simulink model "kamerol"  (R2021b)
settings: Solver=VariableStepAuto  StartTime=0.0  StopTime=10.0  RelTol=1e-3
undefined symbols (not defined in the file): admireDB
libraries: simulink_extras x104, simulink x24, sharedutil x1
(part 6 of 14)

== system kamerol/Aerodynamics/RollMomentCoefficient/MachRegion4/Crmp ==
  in_bus : Inport
  Bus Selector : BusSelector  OutputSignals=AeroIn_Bus.angleOfAttack_deg,AeroIn_Bus.mach_nd,AeroIn_Bus.pc,AeroIn_Bus.qacorr
  Crmp_ : Subsystem
  Crmp : Outport
  wires:
  Bus Selector/4 -> Crmp_/4(qacorr)  "<qacorr>"
  Bus Selector/3 -> Crmp_/3(pc)  "<pc>"
  Bus Selector/2 -> Crmp_/2(mach_nd)  "<mach_nd>"
  Bus Selector/1 -> Crmp_/1(angleOfAttack_deg)  "<angleOfAttack_deg>"
  Crmp_/1(Crmp) -> Crmp/1
  in_bus/1 -> Bus Selector/1  "in_bus"

== system kamerol/Aerodynamics/RollMomentCoefficient/MachRegion4/Crmpbeta ==
  Crmpbeta_ : Constant  Value=0
  Crmpbeta : Outport
  wires:
  Crmpbeta_/1 -> Crmpbeta/1

== system kamerol/Aerodynamics/RollMomentCoefficient/MachRegion4/Crmr ==
  in_bus : Inport
  Bus Selector : BusSelector  OutputSignals=AeroIn_Bus.angleOfAttack_deg,AeroIn_Bus.mach_nd,AeroIn_Bus.rc
  Crmr_ : Subsystem
  Crmr : Outport
  wires:
  Bus Selector/3 -> Crmr_/3(rc)  "<rc>"
  Bus Selector/2 -> Crmr_/2(mach_nd)  "<mach_nd>"
  Bus Selector/1 -> Crmr_/1(angleOfAttack_deg)  "<angleOfAttack_deg>"
  Crmr_/1(Crmr) -> Crmr/1
  in_bus/1 -> Bus Selector/1  "in_bus"

== system kamerol/Aerodynamics/RollMomentCoefficient/MachRegion4/Crmrbeta ==
  Crmrbeta_ : Constant  Value=0
  Crmrbeta : Outport
  wires:
  Crmrbeta_/1 -> Crmrbeta/1

== system kamerol/Aerodynamics/RollMomentCoefficient/MachRegion4/Crmrde ==
  in_bus : Inport
  Bus Selector : BusSelector  OutputSignals=AeroIn_Bus.mach_nd,AeroIn_Bus.angleOfAttack_deg,AeroIn_Bus.rc,AeroIn_Bus.dEI,eieff,AeroIn_Bus.dEY,eoeff
  Crmrde_ : Subsystem
  Crmrde : Outport
  wires:
  Bus Selector/1 -> Crmrde_/1(mach_nd)  "<mach_nd>"
  Bus Selector/2 -> Crmrde_/2(angleOfAttack_deg)  "<angleOfAttack_deg>"
  Bus Selector/3 -> Crmrde_/3(rc)  "<rc>"
  Bus Selector/4 -> Crmrde_/4(dEI)  "<dEI>"
  Bus Selector/5 -> Crmrde_/5(eieff)  "<eieff>"
  Bus Selector/6 -> Crmrde_/6(dEY)  "<dEY>"
  Bus Selector/7 -> Crmrde_/7(eoeff)  "<eoeff>"
  Crmrde_/1(Crmrde) -> Crmrde/1
  in_bus/1 -> Bus Selector/1  "in_bus"

== system kamerol/Aerodynamics/RollMomentCoefficient/MachRegion4/eoeff1 ==
  AeroIn_Bus : Inport
  Bus Selector : BusSelector  OutputSignals=mach_nd
  CRMDAYOD_M : Lookup_n-D  NumberOfTableDimensions=1  BreakpointsForDimension1=admireDB.aerodata_asym_ext.CRMDAYOD.breakpoints.M  BreakpointsForDimension3=[5, 7]  Table=admireDB.aerodata_asym_ext.CRMDAYOD.newTable  ExtrapMethod=Clip  InternalRulePriority=Speed  RndMeth=Simplest  InputSameDT=on
  Constant : Constant
  Sum : Sum  Inputs=-+|
  eoeff : Outport
  eieff : Outport  Port=2
  wires:
  Sum/1 -> eieff/1
  CRMDAYOD_M/1 -> eoeff/1, Sum/1
  Constant/1 -> Sum/2
  Bus Selector/1 -> CRMDAYOD_M/1  "<mach_nd>"
  AeroIn_Bus/1 -> Bus Selector/1

== system kamerol/Aerodynamics/TangentialForceCoefficient/MachRegion1/Ctalfa ==
  in_bus : Inport
  Bus Selector : BusSelector  OutputSignals=AeroIn_Bus.angleOfAttack_deg
  CTAL_ALFA : Lookup_n-D  NumberOfTableDimensions=1  BreakpointsForDimension1=admireDB.aerodata_sym.CTAL.breakpoints.ALFA  BreakpointsForDimension3=[5, 7]  Table=admireDB.aerodata_sym.CTAL.newTable  ExtrapMethod=Clip  InternalRulePriority=Speed  RndMeth=Simplest  InputSameDT=on
  Ctalfa : Outport
  wires:
  Bus Selector/1 -> CTAL_ALFA/1  "<angleOfAttack_deg>"
  in_bus/1 -> Bus Selector/1
  CTAL_ALFA/1 -> Ctalfa/1  "Ctalfa"

== system kamerol/Aerodynamics/TangentialForceCoefficient/MachRegion1/Ctbasic ==
  in_bus : Inport
  Bus Selector : BusSelector  OutputSignals=AeroIn_Bus.mach_nd,AeroIn_Bus.altitude_m
  CTH_H_M : Lookup_n-D  BreakpointsForDimension1=admireDB.aerodata_sym.CTH.breakpoints.M  BreakpointsForDimension2=admireDB.aerodata_sym.CTH.breakpoints.H  BreakpointsForDimension3=[5, 7]  Table=admireDB.aerodata_sym.CTH.newTable  ExtrapMethod=Clip  InternalRulePriority=Speed  RndMeth=Simplest  InputSameDT=on
      settings: InputPortMap=u0,u1
  CTZERO_M : Lookup_n-D  NumberOfTableDimensions=1  BreakpointsForDimension1=admireDB.aerodata_sym.CTZERO.breakpoints.M  BreakpointsForDimension3=[5, 7]  Table=admireDB.aerodata_sym.CTZERO.newTable  ExtrapMethod=Clip  InternalRulePriority=Speed  RndMeth=Simplest  InputSameDT=on
  Constant : Constant  Value=1/1000
  Product : Product
  Sum1 : Sum  Inputs=|++
  Ctbasic : Outport
  wires:
  Sum1/1 -> Ctbasic/1
  CTZERO_M/1 -> Sum1/1
  CTH_H_M/1 -> Sum1/2
  Constant/1 -> Product/2
  Product/1 -> CTH_H_M/2
  Bus Selector/2 -> Product/1  "<altitude_m>"
  Bus Selector/1 -> CTZERO_M/1, CTH_H_M/1  "<mach_nd>"
  in_bus/1 -> Bus Selector/1  "in_bus"

== system kamerol/Aerodynamics/TangentialForceCoefficient/MachRegion1/Ctbeta ==
  in_bus : Inport
  Abs : Abs
  Bus Selector : BusSelector  OutputSignals=AeroIn_Bus.angleOfAttack_deg,AeroIn_Bus.dN,AeroIn_Bus.angleOfSideslip_deg
  CTBETA_DN_ALFA : Lookup_n-D  BreakpointsForDimension1=admireDB.aerodata_sym.CTBETA.breakpoints.ALFA  BreakpointsForDimension2=admireDB.aerodata_sym.CTBETA.breakpoints.DN  BreakpointsForDimension3=[5, 7]  Table=admireDB.aerodata_sym.CTBETA.newTable  ExtrapMethod=Clip  InternalRulePriority=Speed  RndMeth=Simplest  InputSameDT=on
      settings: InputPortMap=u0,u1
  CTKB_BETA : Lookup_n-D  NumberOfTableDimensions=1  BreakpointsForDimension1=admireDB.aerodata_sym.CTKB.breakpoints.BETA  BreakpointsForDimension3=[5, 7]  Table=admireDB.aerodata_sym.CTKB.newTable  ExtrapMethod=Clip  InternalRulePriority=Speed  RndMeth=Simplest  InputSameDT=on
  Product : Product
  Ctbeta : Outport
  wires:
  Product/1 -> Ctbeta/1
  CTBETA_DN_ALFA/1 -> Product/1
  CTKB_BETA/1 -> Product/2
  Abs/1 -> CTKB_BETA/1
  Bus Selector/3 -> Abs/1  "<angleOfSideslip_deg>"
  Bus Selector/1 -> CTBETA_DN_ALFA/1  "<angleOfAttack_deg>"
  Bus Selector/2 -> CTBETA_DN_ALFA/2  "<dN>"
  in_bus/1 -> Bus Selector/1

== system kamerol/Aerodynamics/TangentialForceCoefficient/MachRegion1/Ctda ==
  in_bus : Inport
  Abs : Abs
  Abs1 : Abs
  Abs2 : Abs
  Bus Selector : BusSelector  OutputSignals=AeroIn_Bus.angleOfAttack_deg,AeroIn_Bus.dAI,AeroIn_Bus.dAY
  Bus Selector1 : BusSelector  OutputSignals=eieff,eoeff
  CTDAAL_DA_ALFA : Lookup_n-D  BreakpointsForDimension1=admireDB.aerodata_sym.CTDAAL.breakpoints.ALFA  BreakpointsForDimension2=admireDB.aerodata_sym.CTDAAL.breakpoints.DA  BreakpointsForDimension3=[5, 7]  Table=admireDB.aerodata_sym.CTDAAL.newTable  ExtrapMethod=Clip  InternalRulePriority=Speed  RndMeth=Simplest  InputSameDT=on
      settings: InputPortMap=u0,u1
  CTDAAL_DA_ALFA1 : Lookup_n-D  BreakpointsForDimension1=admireDB.aerodata_sym.CTDAAL.breakpoints.ALFA  BreakpointsForDimension2=admireDB.aerodata_sym.CTDAAL.breakpoints.DA  BreakpointsForDimension3=[5, 7]  Table=admireDB.aerodata_sym.CTDAAL.newTable  ExtrapMethod=Clip  InternalRulePriority=Speed  RndMeth=Simplest  InputSameDT=on
      settings: InputPortMap=u0,u1
  Product : Product
  Product1 : Product
  Sum : Sum  Inputs=|++
  Ctda : Outport
  wires:
  Sum/1 -> Ctda/1
  Product1/1 -> Sum/2
  Product/1 -> Sum/1
  Bus Selector1/2 -> Product1/1  "<eoeff>"
  CTDAAL_DA_ALFA1/1 -> Product1/2
  Bus Selector1/1 -> Product/1  "<eieff>"
  CTDAAL_DA_ALFA/1 -> Product/2
  Abs2/1 -> CTDAAL_DA_ALFA1/2
  Abs1/1 -> CTDAAL_DA_ALFA/2
  Abs/1 -> CTDAAL_DA_ALFA/1, CTDAAL_DA_ALFA1/1
  Bus Selector/2 -> Abs1/1  "<dAI>"
  Bus Selector/1 -> Abs/1  "<angleOfAttack_deg>"
  in_bus/1 -> Bus Selector/1, Bus Selector1/1
  Bus Selector/3 -> Abs2/1  "<dAY>"

== system kamerol/Aerodynamics/TangentialForceCoefficient/MachRegion1/Ctdedn ==
  in_bus : Inport
  Bus Selector : BusSelector  OutputSignals=AeroIn_Bus.angleOfAttack_deg,AeroIn_Bus.dE,AeroIn_Bus.dN
  CTDNDE_ALFA_DE_DN : Lookup_n-D  NumberOfTableDimensions=3  BreakpointsForDimension1=admireDB.aerodata_sym.CTDNDE.breakpoints.ALFA  BreakpointsForDimension2=admireDB.aerodata_sym.CTDNDE.breakpoints.DE  BreakpointsForDimension3=admireDB.aerodata_sym.CTDNDE.breakpoints.DN  Table=admireDB.aerodata_sym.CTDNDE.newTable  ExtrapMethod=Clip  InternalRulePriority=Speed  RndMeth=Simplest  InputSameDT=on
      settings: InputPortMap=u0,u1,u2
  Ctdedn : Outport
  wires:
  Bus Selector/1 -> CTDNDE_ALFA_DE_DN/1  "<angleOfAttack_deg>"
  Bus Selector/3 -> CTDNDE_ALFA_DE_DN/3  "<dN>"
  CTDNDE_ALFA_DE_DN/1 -> Ctdedn/1
  Bus Selector/2 -> CTDNDE_ALFA_DE_DN/2  "<dE>"
  in_bus/1 -> Bus Selector/1

== system kamerol/Aerodynamics/TangentialForceCoefficient/MachRegion1/Ctdei ==
  in_bus : Inport
  Bus Selector : BusSelector  OutputSignals=AeroIn_Bus.angleOfAttack_deg,AeroIn_Bus.dEI,eieff
  CTDEAL_DE_ALFA : Lookup_n-D  BreakpointsForDimension1=admireDB.aerodata_sym.CTDEAL.breakpoints.ALFA  BreakpointsForDimension2=admireDB.aerodata_sym.CTDEAL.breakpoints.DE  BreakpointsForDimension3=[5, 7]  Table=admireDB.aerodata_sym.CTDEAL.newTable  ExtrapMethod=Clip  InternalRulePriority=Speed  RndMeth=Simplest  InputSameDT=on
      settings: InputPortMap=u0,u1
  Product : Product
  Ctdei : Outport
  wires:
  Product/1 -> Ctdei/1
  Bus Selector/3 -> Product/2  "<eieff>"
  CTDEAL_DE_ALFA/1 -> Product/1
  Bus Selector/1 -> CTDEAL_DE_ALFA/1  "<angleOfAttack_deg>"
  Bus Selector/2 -> CTDEAL_DE_ALFA/2  "<dEI>"
  in_bus/1 -> Bus Selector/1

== system kamerol/Aerodynamics/TangentialForceCoefficient/MachRegion1/Ctdey ==
  in_bus : Inport
  Bus Selector : BusSelector  OutputSignals=AeroIn_Bus.angleOfAttack_deg,AeroIn_Bus.dEY,eoeff
  CTDEAL_DE_ALFA : Lookup_n-D  BreakpointsForDimension1=admireDB.aerodata_sym.CTDEAL.breakpoints.ALFA  BreakpointsForDimension2=admireDB.aerodata_sym.CTDEAL.breakpoints.DE  BreakpointsForDimension3=[5, 7]  Table=admireDB.aerodata_sym.CTDEAL.newTable  ExtrapMethod=Clip  InternalRulePriority=Speed  RndMeth=Simplest  InputSameDT=on
      settings: InputPortMap=u0,u1
  Product : Product
  Ctdey : Outport
  wires:
  in_bus/1 -> Bus Selector/1
  Bus Selector/2 -> CTDEAL_DE_ALFA/2  "<dEY>"
  Bus Selector/1 -> CTDEAL_DE_ALFA/1  "<angleOfAttack_deg>"
  CTDEAL_DE_ALFA/1 -> Product/1
  Bus Selector/3 -> Product/2  "<eoeff>"
  Product/1 -> Ctdey/1

== system kamerol/Aerodynamics/TangentialForceCoefficient/MachRegion1/Ctdle ==
  in_bus : Inport
  Bus Selector : BusSelector  OutputSignals=AeroIn_Bus.angleOfAttack_deg,AeroIn_Bus.lef_deg,AeroIn_Bus.dN
  CTDLEAL_DLE_ALFA : Lookup_n-D  BreakpointsForDimension1=admireDB.aerodata_sym.CTDLEAL.breakpoints.ALFA  BreakpointsForDimension2=admireDB.aerodata_sym.CTDLEAL.breakpoints.DLE  BreakpointsForDimension3=[5, 7]  Table=admireDB.aerodata_sym.CTDLEAL.newTable  ExtrapMethod=Clip  InternalRulePriority=Speed  RndMeth=Simplest  InputSameDT=on
      settings: InputPortMap=u0,u1
  CTLEDNAL_DN_ALFA : Lookup_n-D  BreakpointsForDimension1=admireDB.aerodata_sym.CTLEDNAL.breakpoints.ALFA  BreakpointsForDimension2=admireDB.aerodata_sym.CTLEDNAL.breakpoints.DN  BreakpointsForDimension3=[5, 7]  Table=admireDB.aerodata_sym.CTLEDNAL.newTable  ExtrapMethod=Clip  InternalRulePriority=Speed  RndMeth=Simplest  InputSameDT=on
      settings: InputPortMap=u0,u1
  Constant : Constant  Value=1/27
  Product : Product  Inputs=3
  Sum : Sum  Inputs=|++
  Ctdle : Outport
  wires:
  Product/1 -> Sum/2
  Constant/1 -> Product/3
  CTLEDNAL_DN_ALFA/1 -> Product/1
  Bus Selector/3 -> CTLEDNAL_DN_ALFA/2  "<dN>"
  Sum/1 -> Ctdle/1
  Bus Selector/1 -> CTLEDNAL_DN_ALFA/1, CTDLEAL_DLE_ALFA/1  "<angleOfAttack_deg>"
  Bus Selector/2 -> Product/2, CTDLEAL_DLE_ALFA/2  "<lef_deg>"
  CTDLEAL_DLE_ALFA/1 -> Sum/1
  in_bus/1 -> Bus Selector/1

== system kamerol/Aerodynamics/TangentialForceCoefficient/MachRegion1/Ctdn ==
  in_bus : Inport
  Bus Selector : BusSelector  OutputSignals=AeroIn_Bus.angleOfAttack_deg,AeroIn_Bus.dN
  CTDNAL_DN_ALFA : Lookup_n-D  BreakpointsForDimension1=admireDB.aerodata_sym.CTDNAL.breakpoints.ALFA  BreakpointsForDimension2=admireDB.aerodata_sym.CTDNAL.breakpoints.DN  BreakpointsForDimension3=[5, 7]  Table=admireDB.aerodata_sym.CTDNAL.newTable  ExtrapMethod=Clip  InternalRulePriority=Speed  RndMeth=Simplest  InputSameDT=on
      settings: InputPortMap=u0,u1
  Ctdn : Outport
  wires:
  in_bus/1 -> Bus Selector/1
  CTDNAL_DN_ALFA/1 -> Ctdn/1
  Bus Selector/2 -> CTDNAL_DN_ALFA/2  "<dN>"
  Bus Selector/1 -> CTDNAL_DN_ALFA/1  "<angleOfAttack_deg>"

== system kamerol/Aerodynamics/TangentialForceCoefficient/MachRegion1/Ctdr ==
  in_bus : Inport
  Abs : Abs
  Bus Selector : BusSelector  OutputSignals=AeroIn_Bus.mach_nd,AeroIn_Bus.rud_deg
  CTMDR_DR_M : Lookup_n-D  BreakpointsForDimension1=admireDB.aerodata_sym.CTMDR.breakpoints.M  BreakpointsForDimension2=admireDB.aerodata_sym.CTMDR.breakpoints.DR  BreakpointsForDimension3=[5, 7]  Table=admireDB.aerodata_sym.CTMDR.newTable  ExtrapMethod=Clip  InternalRulePriority=Speed  RndMeth=Simplest  InputSameDT=on
      settings: InputPortMap=u0,u1
  Ctdr : Outport
  wires:
  Abs/1 -> CTMDR_DR_M/2
  Bus Selector/1 -> CTMDR_DR_M/1  "<mach_nd>"
  Bus Selector/2 -> Abs/1  "<rud_deg>"
  in_bus/1 -> Bus Selector/1
  CTMDR_DR_M/1 -> Ctdr/1

== system kamerol/Aerodynamics/TangentialForceCoefficient/MachRegion1/Cthigh ==
  in_bus : Inport
  Bus Selector : BusSelector  OutputSignals=AeroIn_Bus.angleOfAttack_deg,AeroIn_Bus.dN,AeroIn_Bus.dE
  CTHDE_DE_ALFA : Lookup_n-D  BreakpointsForDimension1=admireDB.aerodata_high.CTHDE.breakpoints.ALFA  BreakpointsForDimension2=admireDB.aerodata_high.CTHDE.breakpoints.DE  BreakpointsForDimension3=[5, 7]  Table=admireDB.aerodata_high.CTHDE.newTable  ExtrapMethod=Clip  InternalRulePriority=Speed  RndMeth=Simplest  InputSameDT=on
      settings: InputPortMap=u0,u1
  CTHDN_DN_ALFA : Lookup_n-D  BreakpointsForDimension1=admireDB.aerodata_high.CTHDN.breakpoints.ALFA  BreakpointsForDimension2=admireDB.aerodata_high.CTHDN.breakpoints.DN  BreakpointsForDimension3=[5, 7]  Table=admireDB.aerodata_high.CTHDN.newTable  ExtrapMethod=Clip  InternalRulePriority=Speed  RndMeth=Simplest  InputSameDT=on
      settings: InputPortMap=u0,u1
  CTHZERO_ALFA : Lookup_n-D  NumberOfTableDimensions=1  BreakpointsForDimension1=admireDB.aerodata_high.CTHZERO.breakpoints.ALFA  BreakpointsForDimension3=[5, 7]  Table=admireDB.aerodata_high.CTHZERO.newTable  ExtrapMethod=Clip  InternalRulePriority=Speed  RndMeth=Simplest  InputSameDT=on
  Sum : Sum  Inputs=+++
  Cthigh : Outport
  wires:
  CTHZERO_ALFA/1 -> Sum/1
  CTHDE_DE_ALFA/1 -> Sum/3
  CTHDN_DN_ALFA/1 -> Sum/2
  Bus Selector/3 -> CTHDE_DE_ALFA/2  "<dE>"
  Bus Selector/2 -> CTHDN_DN_ALFA/2  "<dN>"
  Sum/1 -> Cthigh/1
  in_bus/1 -> Bus Selector/1
  Bus Selector/1 -> CTHZERO_ALFA/1, CTHDN_DN_ALFA/1, CTHDE_DE_ALFA/1  "<angleOfAttack_deg>"

== system kamerol/Aerodynamics/TangentialForceCoefficient/MachRegion1/Ctlg ==
  in_bus : Inport
  Abs : Abs
  Bus Selector : BusSelector  OutputSignals=AeroIn_Bus.angleOfAttack_deg,AeroIn_Bus.angleOfSideslip_deg,AeroIn_Bus.lg_bool
  CTLST_BETA_ALFA : Lookup_n-D  BreakpointsForDimension1=admireDB.aerodata_sym.CTLST.breakpoints.ALFA  BreakpointsForDimension2=admireDB.aerodata_sym.CTLST.breakpoints.BETA  BreakpointsForDimension3=[5, 7]  Table=admireDB.aerodata_sym.CTLST.newTable  ExtrapMethod=Clip  InternalRulePriority=Speed  RndMeth=Simplest  InputSameDT=on
      settings: InputPortMap=u0,u1
  Product : Product  Inputs=**
  Ctlg : Outport
  wires:
  Abs/1 -> CTLST_BETA_ALFA/2
  Bus Selector/3 -> Product/2  "<lg_bool>"
  CTLST_BETA_ALFA/1 -> Product/1
  in_bus/1 -> Bus Selector/1
  Bus Selector/2 -> Abs/1  "<angleOfSideslip_deg>"
  Bus Selector/1 -> CTLST_BETA_ALFA/1  "<angleOfAttack_deg>"
  Product/1 -> Ctlg/1

== system kamerol/Aerodynamics/TangentialForceCoefficient/MachRegion1/eoeff ==
  AeroIn_Bus : Inport
  Bus Selector : BusSelector  OutputSignals=mach_nd
  CTDEYODE_M : Lookup_n-D  NumberOfTableDimensions=1  BreakpointsForDimension1=admireDB.aerodata_sym.CTDEYODE.breakpoints.M  BreakpointsForDimension3=[5, 7]  Table=admireDB.aerodata_sym.CTDEYODE.newTable  ExtrapMethod=Clip  InternalRulePriority=Speed  RndMeth=Simplest  InputSameDT=on
  Constant : Constant
  Sum : Sum  Inputs=-+|
  eoeff : Outport
  eieff : Outport  Port=2
  wires:
  Sum/1 -> eieff/1
  CTDEYODE_M/1 -> eoeff/1, Sum/1
  Constant/1 -> Sum/2
  Bus Selector/1 -> CTDEYODE_M/1  "<mach_nd>"
  AeroIn_Bus/1 -> Bus Selector/1

== system kamerol/Aerodynamics/TangentialForceCoefficient/MachRegion2/Ctalfa ==
  in_bus : Inport
  Bus Selector : BusSelector  OutputSignals=AeroIn_Bus.angleOfAttack_deg,AeroIn_Bus.tflow,AeroIn_Bus.tfhigh
  CTAL_ALFA : Lookup_n-D  NumberOfTableDimensions=1  BreakpointsForDimension1=admireDB.aerodata_sym.CTAL.breakpoints.ALFA  BreakpointsForDimension3=[5, 7]  Table=admireDB.aerodata_sym.CTAL.newTable  ExtrapMethod=Clip  InternalRulePriority=Speed  RndMeth=Simplest  InputSameDT=on
  CTMA_M_ALFA : Lookup_n-D  BreakpointsForDimension1=admireDB.aerodata_sym.CTMA.breakpoints.ALFA  BreakpointsForDimension2=admireDB.aerodata_sym.CTMA.breakpoints.M  BreakpointsForDimension3=[5, 7]  Table=admireDB.aerodata_sym.CTMA.newTable  ExtrapMethod=Clip  InternalRulePriority=Speed  RndMeth=Simplest  InputSameDT=on
      settings: InputPortMap=u0,u1
  Constant : Constant  Value=0.5
  Product : Product
  Product1 : Product
  Sum : Sum  Inputs=|++
  Ctalfa : Outport
  wires:
  Bus Selector/3 -> Product1/1  "<tfhigh>"
  Bus Selector/2 -> Product/2  "<tflow>"
  Product1/1 -> Sum/2
  CTMA_M_ALFA/1 -> Product1/2
  Sum/1 -> Ctalfa/1
  Product/1 -> Sum/1
  Constant/1 -> CTMA_M_ALFA/2
  CTAL_ALFA/1 -> Product/1  "Ctalfa"
  in_bus/1 -> Bus Selector/1
  Bus Selector/1 -> CTAL_ALFA/1, CTMA_M_ALFA/1  "<angleOfAttack_deg>"

== system kamerol/Aerodynamics/TangentialForceCoefficient/MachRegion2/Ctbasic ==
  in_bus : Inport
  Bus Selector : BusSelector  OutputSignals=AeroIn_Bus.mach_nd,AeroIn_Bus.altitude_m
  CTH_H_M : Lookup_n-D  BreakpointsForDimension1=admireDB.aerodata_sym.CTH.breakpoints.M  BreakpointsForDimension2=admireDB.aerodata_sym.CTH.breakpoints.H  BreakpointsForDimension3=[5, 7]  Table=admireDB.aerodata_sym.CTH.newTable  ExtrapMethod=Clip  InternalRulePriority=Speed  RndMeth=Simplest  InputSameDT=on
      settings: InputPortMap=u0,u1
  CTZERO_M : Lookup_n-D  NumberOfTableDimensions=1  BreakpointsForDimension1=admireDB.aerodata_sym.CTZERO.breakpoints.M  BreakpointsForDimension3=[5, 7]  Table=admireDB.aerodata_sym.CTZERO.newTable  ExtrapMethod=Clip  InternalRulePriority=Speed  RndMeth=Simplest  InputSameDT=on
  Constant : Constant  Value=1/1000
  Product : Product
  Sum1 : Sum  Inputs=|++
  Ctbasic : Outport
  wires:
  CTH_H_M/1 -> Sum1/2
  Constant/1 -> Product/2
  Bus Selector/2 -> Product/1  "<altitude_m>"
  Product/1 -> CTH_H_M/2
  CTZERO_M/1 -> Sum1/1
  Bus Selector/1 -> CTZERO_M/1, CTH_H_M/1  "<mach_nd>"
  in_bus/1 -> Bus Selector/1  "in_bus"
  Sum1/1 -> Ctbasic/1

== system kamerol/Aerodynamics/TangentialForceCoefficient/MachRegion2/Ctbeta ==
  in_bus : Inport
  Abs : Abs
  Bus Selector : BusSelector  OutputSignals=AeroIn_Bus.angleOfAttack_deg,AeroIn_Bus.dN,AeroIn_Bus.tflow,AeroIn_Bus.angleOfSideslip_deg
  CTBETA_DN_ALFA : Lookup_n-D  BreakpointsForDimension1=admireDB.aerodata_sym.CTBETA.breakpoints.ALFA  BreakpointsForDimension2=admireDB.aerodata_sym.CTBETA.breakpoints.DN  BreakpointsForDimension3=[5, 7]  Table=admireDB.aerodata_sym.CTBETA.newTable  ExtrapMethod=Clip  InternalRulePriority=Speed  RndMeth=Simplest  InputSameDT=on
      settings: InputPortMap=u0,u1
  CTKB_BETA : Lookup_n-D  NumberOfTableDimensions=1  BreakpointsForDimension1=admireDB.aerodata_sym.CTKB.breakpoints.BETA  BreakpointsForDimension3=[5, 7]  Table=admireDB.aerodata_sym.CTKB.newTable  ExtrapMethod=Clip  InternalRulePriority=Speed  RndMeth=Simplest  InputSameDT=on
  Product : Product  Inputs=3
  Ctbeta : Outport
  wires:
  Bus Selector/3 -> Product/2  "<tflow>"
  in_bus/1 -> Bus Selector/1
  Bus Selector/2 -> CTBETA_DN_ALFA/2  "<dN>"
  Bus Selector/1 -> CTBETA_DN_ALFA/1  "<angleOfAttack_deg>"
  Bus Selector/4 -> Abs/1  "<angleOfSideslip_deg>"
  Abs/1 -> CTKB_BETA/1
  CTKB_BETA/1 -> Product/3
  CTBETA_DN_ALFA/1 -> Product/1
  Product/1 -> Ctbeta/1

== system kamerol/Aerodynamics/TangentialForceCoefficient/MachRegion2/Ctda ==
  in_bus : Inport
  Abs : Abs
  Abs1 : Abs
  Abs2 : Abs
  Bus Selector : BusSelector  OutputSignals=AeroIn_Bus.angleOfAttack_deg,AeroIn_Bus.dAI,AeroIn_Bus.dAY
  Bus Selector1 : BusSelector  OutputSignals=AeroIn_Bus.tflow,eiefflow,eoefflow,eieffhigh,eoeffhigh,AeroIn_Bus.tfhigh
  CTDAAL_DA_ALFA : Lookup_n-D  BreakpointsForDimension1=admireDB.aerodata_sym.CTDAAL.breakpoints.ALFA  BreakpointsForDimension2=admireDB.aerodata_sym.CTDAAL.breakpoints.DA  BreakpointsForDimension3=[5, 7]  Table=admireDB.aerodata_sym.CTDAAL.newTable  ExtrapMethod=Clip  InternalRulePriority=Speed  RndMeth=Simplest  InputSameDT=on
      settings: InputPortMap=u0,u1
  CTDAAL_DA_ALFA1 : Lookup_n-D  BreakpointsForDimension1=admireDB.aerodata_sym.CTDAAL.breakpoints.ALFA  BreakpointsForDimension2=admireDB.aerodata_sym.CTDAAL.breakpoints.DA  BreakpointsForDimension3=[5, 7]  Table=admireDB.aerodata_sym.CTDAAL.newTable  ExtrapMethod=Clip  InternalRulePriority=Speed  RndMeth=Simplest  InputSameDT=on
      settings: InputPortMap=u0,u1
  CTDAM_DA_M : Lookup_n-D  BreakpointsForDimension1=admireDB.aerodata_sym.CTDAM.breakpoints.M  BreakpointsForDimension2=admireDB.aerodata_sym.CTDAM.breakpoints.DA  BreakpointsForDimension3=[5, 7]  Table=admireDB.aerodata_sym.CTDAM.newTable  ExtrapMethod=Clip  InternalRulePriority=Speed  RndMeth=Simplest  InputSameDT=on
      settings: InputPortMap=u0,u1
  CTDAM_DA_M1 : Lookup_n-D  BreakpointsForDimension1=admireDB.aerodata_sym.CTDAM.breakpoints.M  BreakpointsForDimension2=admireDB.aerodata_sym.CTDAM.breakpoints.DA  BreakpointsForDimension3=[5, 7]  Table=admireDB.aerodata_sym.CTDAM.newTable  ExtrapMethod=Clip  InternalRulePriority=Speed  RndMeth=Simplest  InputSameDT=on
      settings: InputPortMap=u0,u1
  Product{,1..5} (6 alike) : Product
  Sum : Sum  Inputs=|++
  Sum1 : Sum  Inputs=++|
  Sum2 : Sum  Inputs=|++
  mach_nd_cnst : Constant  Value=0.5
  Ctda : Outport
  wires:
  Product5/1 -> Sum1/2
  Bus Selector1/6 -> Product5/1  "<tfhigh>"
  Sum2/1 -> Product5/2
  Product3/1 -> Sum2/2
  Product4/1 -> Sum2/1
  Bus Selector1/5 -> Product3/1  "<eoeffhigh>"
  Bus Selector1/4 -> Product4/1  "<eieffhigh>"
  CTDAM_DA_M/1 -> Product4/2
  CTDAM_DA_M1/1 -> Product3/2
  mach_nd_cnst/1 -> CTDAM_DA_M/1, CTDAM_DA_M1/1
  Sum1/1 -> Ctda/1
  Product2/1 -> Sum1/1
  Bus Selector1/1 -> Product2/1  "<tflow>"
  Bus Selector/3 -> Abs2/1  "<dAY>"
  in_bus/1 -> Bus Selector1/1, Bus Selector/1
  Bus Selector/1 -> Abs/1  "<angleOfAttack_deg>"
  Bus Selector/2 -> Abs1/1  "<dAI>"
  Abs/1 -> CTDAAL_DA_ALFA/1, CTDAAL_DA_ALFA1/1
  Abs1/1 -> CTDAAL_DA_ALFA/2, CTDAM_DA_M/2
  Abs2/1 -> CTDAAL_DA_ALFA1/2, CTDAM_DA_M1/2
  CTDAAL_DA_ALFA/1 -> Product/2
  Bus Selector1/2 -> Product/1  "<eiefflow>"
  CTDAAL_DA_ALFA1/1 -> Product1/2
  Bus Selector1/3 -> Product1/1  "<eoefflow>"
  Product/1 -> Sum/1
  Product1/1 -> Sum/2
  Sum/1 -> Product2/2

== system kamerol/Aerodynamics/TangentialForceCoefficient/MachRegion2/Ctdedn ==
  in_bus : Inport
  Bus Selector : BusSelector  OutputSignals=AeroIn_Bus.angleOfAttack_deg,AeroIn_Bus.dE,AeroIn_Bus.dN,AeroIn_Bus.tflow
  CTDNDE_ALFA_DE_DN1 : Lookup_n-D  NumberOfTableDimensions=3  BreakpointsForDimension1=admireDB.aerodata_sym.CTDNDE.breakpoints.ALFA  BreakpointsForDimension2=admireDB.aerodata_sym.CTDNDE.breakpoints.DE  BreakpointsForDimension3=admireDB.aerodata_sym.CTDNDE.breakpoints.DN  Table=admireDB.aerodata_sym.CTDNDE.newTable  ExtrapMethod=Clip  InternalRulePriority=Speed  RndMeth=Simplest  InputSameDT=on
      settings: InputPortMap=u0,u1,u2
  Product : Product
  Ctdedn : Outport
  wires:
  Bus Selector/4 -> Product/2  "<tflow>"
  Product/1 -> Ctdedn/1
  Bus Selector/1 -> CTDNDE_ALFA_DE_DN1/1  "<angleOfAttack_deg>"
  Bus Selector/3 -> CTDNDE_ALFA_DE_DN1/3  "<dN>"
  Bus Selector/2 -> CTDNDE_ALFA_DE_DN1/2  "<dE>"
  in_bus/1 -> Bus Selector/1
  CTDNDE_ALFA_DE_DN1/1 -> Product/1

== system kamerol/Aerodynamics/TangentialForceCoefficient/MachRegion2/Ctdei ==
  in_bus : Inport
  Bus Selector : BusSelector  OutputSignals=AeroIn_Bus.angleOfAttack_deg,AeroIn_Bus.dEI,eiefflow,AeroIn_Bus.tflow,eieffhigh,AeroIn_Bus.tfhigh
  CTDEAL_DE_ALFA1 : Lookup_n-D  BreakpointsForDimension1=admireDB.aerodata_sym.CTDEAL.breakpoints.ALFA  BreakpointsForDimension2=admireDB.aerodata_sym.CTDEAL.breakpoints.DE  BreakpointsForDimension3=[5, 7]  Table=admireDB.aerodata_sym.CTDEAL.newTable  ExtrapMethod=Clip  InternalRulePriority=Speed  RndMeth=Simplest  InputSameDT=on
      settings: InputPortMap=u0,u1
  CTMDEA_ALFA_DE_M : Lookup_n-D  NumberOfTableDimensions=3  BreakpointsForDimension1=admireDB.aerodata_sym.CTMDEA.breakpoints.ALFA  BreakpointsForDimension2=admireDB.aerodata_sym.CTMDEA.breakpoints.DE  BreakpointsForDimension3=admireDB.aerodata_sym.CTMDEA.breakpoints.M  Table=admireDB.aerodata_sym.CTMDEA.newTable  ExtrapMethod=Clip  InternalRulePriority=Speed  RndMeth=Simplest  InputSameDT=on
      settings: InputPortMap=u0,u1,u2
  Product : Product  Inputs=3
  Product1 : Product  Inputs=3
  Sum : Sum  Inputs=|++
  mach_nd_cnst : Constant  Value=0.5
  Ctdei : Outport
  wires:
  Product1/1 -> Sum/2
  Sum/1 -> Ctdei/1
  Bus Selector/6 -> Product1/2  "<tfhigh>"
  CTMDEA_ALFA_DE_M/1 -> Product1/3
  Bus Selector/5 -> Product1/1  "<eieffhigh>"
  Bus Selector/4 -> Product/3  "<tflow>"
  mach_nd_cnst/1 -> CTMDEA_ALFA_DE_M/3
  in_bus/1 -> Bus Selector/1
  Bus Selector/2 -> CTMDEA_ALFA_DE_M/2, CTDEAL_DE_ALFA1/2  "<dEI>"
  Bus Selector/1 -> CTDEAL_DE_ALFA1/1, CTMDEA_ALFA_DE_M/1  "<angleOfAttack_deg>"
  CTDEAL_DE_ALFA1/1 -> Product/1
  Bus Selector/3 -> Product/2  "<eiefflow>"
  Product/1 -> Sum/1

== system kamerol/Aerodynamics/TangentialForceCoefficient/MachRegion2/Ctdey ==
  in_bus : Inport
  Bus Selector : BusSelector  OutputSignals=AeroIn_Bus.angleOfAttack_deg,AeroIn_Bus.dEY,eoefflow,AeroIn_Bus.tflow,eoeffhigh,AeroIn_Bus.tfhigh
  CTDEAL_DE_ALFA1 : Lookup_n-D  BreakpointsForDimension1=admireDB.aerodata_sym.CTDEAL.breakpoints.ALFA  BreakpointsForDimension2=admireDB.aerodata_sym.CTDEAL.breakpoints.DE  BreakpointsForDimension3=[5, 7]  Table=admireDB.aerodata_sym.CTDEAL.newTable  ExtrapMethod=Clip  InternalRulePriority=Speed  RndMeth=Simplest  InputSameDT=on
      settings: InputPortMap=u0,u1
  CTMDEA_ALFA_DE_M : Lookup_n-D  NumberOfTableDimensions=3  BreakpointsForDimension1=admireDB.aerodata_sym.CTMDEA.breakpoints.ALFA  BreakpointsForDimension2=admireDB.aerodata_sym.CTMDEA.breakpoints.DE  BreakpointsForDimension3=admireDB.aerodata_sym.CTMDEA.breakpoints.M  Table=admireDB.aerodata_sym.CTMDEA.newTable  ExtrapMethod=Clip  InternalRulePriority=Speed  RndMeth=Simplest  InputSameDT=on
      settings: InputPortMap=u0,u1,u2
  Product : Product  Inputs=3
  Product1 : Product  Inputs=3
  Sum : Sum  Inputs=|++
  mach_nd_cnst : Constant  Value=0.5
  Ctdey : Outport
  wires:
  Product/1 -> Sum/1
  Bus Selector/3 -> Product/2  "<eoefflow>"
  CTDEAL_DE_ALFA1/1 -> Product/1
  Bus Selector/1 -> CTDEAL_DE_ALFA1/1, CTMDEA_ALFA_DE_M/1  "<angleOfAttack_deg>"
  Bus Selector/2 -> CTMDEA_ALFA_DE_M/2, CTDEAL_DE_ALFA1/2  "<dEY>"
  in_bus/1 -> Bus Selector/1
  mach_nd_cnst/1 -> CTMDEA_ALFA_DE_M/3
  Bus Selector/4 -> Product/3  "<tflow>"
  Bus Selector/5 -> Product1/1  "<eoeffhigh>"
  CTMDEA_ALFA_DE_M/1 -> Product1/3
  Bus Selector/6 -> Product1/2  "<tfhigh>"
  Sum/1 -> Ctdey/1
  Product1/1 -> Sum/2

== system kamerol/Aerodynamics/TangentialForceCoefficient/MachRegion2/Ctdle ==
  in_bus : Inport
  Bus Selector : BusSelector  OutputSignals=AeroIn_Bus.tflow,AeroIn_Bus.angleOfAttack_deg,AeroIn_Bus.lef_deg,AeroIn_Bus.dN,AeroIn_Bus.tfhigh
  CTDLEAL_DLE_ALFA : Lookup_n-D  BreakpointsForDimension1=admireDB.aerodata_sym.CTDLEAL.breakpoints.ALFA  BreakpointsForDimension2=admireDB.aerodata_sym.CTDLEAL.breakpoints.DLE  BreakpointsForDimension3=[5, 7]  Table=admireDB.aerodata_sym.CTDLEAL.newTable  ExtrapMethod=Clip  InternalRulePriority=Speed  RndMeth=Simplest  InputSameDT=on
      settings: InputPortMap=u0,u1
  CTLEDNAL_DN_ALFA : Lookup_n-D  BreakpointsForDimension1=admireDB.aerodata_sym.CTLEDNAL.breakpoints.ALFA  BreakpointsForDimension2=admireDB.aerodata_sym.CTLEDNAL.breakpoints.DN  BreakpointsForDimension3=[5, 7]  Table=admireDB.aerodata_sym.CTLEDNAL.newTable  ExtrapMethod=Clip  InternalRulePriority=Speed  RndMeth=Simplest  InputSameDT=on
      settings: InputPortMap=u0,u1
  CTMDLEA_ALFA_DLE_M : Lookup_n-D  NumberOfTableDimensions=3  BreakpointsForDimension1=admireDB.aerodata_sym.CTMDLEA.breakpoints.ALFA  BreakpointsForDimension2=admireDB.aerodata_sym.CTMDLEA.breakpoints.DLE  BreakpointsForDimension3=admireDB.aerodata_sym.CTMDLEA.breakpoints.M  Table=admireDB.aerodata_sym.CTMDLEA.newTable  ExtrapMethod=Clip  InternalRulePriority=Speed  RndMeth=Simplest  InputSameDT=on
      settings: InputPortMap=u0,u1,u2
  Constant : Constant  Value=1/27
  Product : Product  Inputs=3
  Product1 : Product
  Product2 : Product
  Sum : Sum  Inputs=|++
  Sum1 : Sum  Inputs=|++
  mach_nd_cnst : Constant  Value=0.5
  Ctdle : Outport
  wires:
  Sum1/1 -> Ctdle/1
  Product2/1 -> Sum1/2
  Product1/1 -> Sum1/1
  Bus Selector/5 -> Product2/1  "<tfhigh>"
  CTMDLEA_ALFA_DLE_M/1 -> Product2/2
  Bus Selector/1 -> Product1/1  "<tflow>"
  mach_nd_cnst/1 -> CTMDLEA_ALFA_DLE_M/3
  in_bus/1 -> Bus Selector/1
  CTDLEAL_DLE_ALFA/1 -> Sum/1
  Bus Selector/3 -> Product/2, CTMDLEA_ALFA_DLE_M/2, CTDLEAL_DLE_ALFA/2  "<lef_deg>"
  Bus Selector/2 -> CTDLEAL_DLE_ALFA/1, CTLEDNAL_DN_ALFA/1, CTMDLEA_ALFA_DLE_M/1  "<angleOfAttack_deg>"
  Sum/1 -> Product1/2
  Bus Selector/4 -> CTLEDNAL_DN_ALFA/2  "<dN>"
  CTLEDNAL_DN_ALFA/1 -> Product/1
  Constant/1 -> Product/3
  Product/1 -> Sum/2

== system kamerol/Aerodynamics/TangentialForceCoefficient/MachRegion2/Ctdn ==
  in_bus : Inport
  Bus Selector : BusSelector  OutputSignals=AeroIn_Bus.angleOfAttack_deg,AeroIn_Bus.dN,AeroIn_Bus.tflow,AeroIn_Bus.tfhigh
  CTDNAL_DN_ALFA : Lookup_n-D  BreakpointsForDimension1=admireDB.aerodata_sym.CTDNAL.breakpoints.ALFA  BreakpointsForDimension2=admireDB.aerodata_sym.CTDNAL.breakpoints.DN  BreakpointsForDimension3=[5, 7]  Table=admireDB.aerodata_sym.CTDNAL.newTable  ExtrapMethod=Clip  InternalRulePriority=Speed  RndMeth=Simplest  InputSameDT=on
      settings: InputPortMap=u0,u1
  CTMDNA_ALFA_DN_M : Lookup_n-D  NumberOfTableDimensions=3  BreakpointsForDimension1=admireDB.aerodata_sym.CTMDNA.breakpoints.ALFA  BreakpointsForDimension2=admireDB.aerodata_sym.CTMDNA.breakpoints.DN  BreakpointsForDimension3=admireDB.aerodata_sym.CTMDNA.breakpoints.M  Table=admireDB.aerodata_sym.CTMDNA.newTable  ExtrapMethod=Clip  InternalRulePriority=Speed  RndMeth=Simplest  InputSameDT=on
      settings: InputPortMap=u0,u1,u2
  Constant : Constant  Value=0.5
  Product : Product  Inputs=**
  Product1 : Product  Inputs=**
  Sum : Sum  Inputs=|++
  Ctdn : Outport
  wires:
  Product1/1 -> Sum/2
  Bus Selector/4 -> Product1/1  "<tfhigh>"
  CTMDNA_ALFA_DN_M/1 -> Product1/2
  Bus Selector/3 -> Product/2  "<tflow>"
  Constant/1 -> CTMDNA_ALFA_DN_M/3
  Product/1 -> Sum/1
  Sum/1 -> Ctdn/1
  Bus Selector/1 -> CTDNAL_DN_ALFA/1, CTMDNA_ALFA_DN_M/1  "<angleOfAttack_deg>"
  Bus Selector/2 -> CTMDNA_ALFA_DN_M/2, CTDNAL_DN_ALFA/2  "<dN>"
  CTDNAL_DN_ALFA/1 -> Product/1
  in_bus/1 -> Bus Selector/1

== system kamerol/Aerodynamics/TangentialForceCoefficient/MachRegion2/Ctdr ==
  in_bus : Inport
  Abs : Abs
  Bus Selector : BusSelector  OutputSignals=AeroIn_Bus.mach_nd,AeroIn_Bus.rud_deg
  CTMDR_DR_M : Lookup_n-D  BreakpointsForDimension1=admireDB.aerodata_sym.CTMDR.breakpoints.M  BreakpointsForDimension2=admireDB.aerodata_sym.CTMDR.breakpoints.DR  BreakpointsForDimension3=[5, 7]  Table=admireDB.aerodata_sym.CTMDR.newTable  ExtrapMethod=Clip  InternalRulePriority=Speed  RndMeth=Simplest  InputSameDT=on
      settings: InputPortMap=u0,u1
  Ctdr : Outport
  wires:
  CTMDR_DR_M/1 -> Ctdr/1
  in_bus/1 -> Bus Selector/1
  Bus Selector/2 -> Abs/1  "<rud_deg>"
  Bus Selector/1 -> CTMDR_DR_M/1  "<mach_nd>"
  Abs/1 -> CTMDR_DR_M/2

== system kamerol/Aerodynamics/TangentialForceCoefficient/MachRegion2/Cthigh ==
  Constant : Constant  Value=0
  Cthigh : Outport
  wires:
  Constant/1 -> Cthigh/1

== system kamerol/Aerodynamics/TangentialForceCoefficient/MachRegion2/Ctlg ==
  in_bus : Inport
  Abs : Abs
  Bus Selector : BusSelector  OutputSignals=AeroIn_Bus.angleOfAttack_deg,AeroIn_Bus.angleOfSideslip_deg,AeroIn_Bus.lg_bool
  CTLST_BETA_ALFA : Lookup_n-D  BreakpointsForDimension1=admireDB.aerodata_sym.CTLST.breakpoints.ALFA  BreakpointsForDimension2=admireDB.aerodata_sym.CTLST.breakpoints.BETA  BreakpointsForDimension3=[5, 7]  Table=admireDB.aerodata_sym.CTLST.newTable  ExtrapMethod=Clip  InternalRulePriority=Speed  RndMeth=Simplest  InputSameDT=on
      settings: InputPortMap=u0,u1
  Product : Product  Inputs=**
  Ctlg : Outport
  wires:
  Product/1 -> Ctlg/1
  Bus Selector/1 -> CTLST_BETA_ALFA/1  "<angleOfAttack_deg>"
  Bus Selector/2 -> Abs/1  "<angleOfSideslip_deg>"
  in_bus/1 -> Bus Selector/1
  CTLST_BETA_ALFA/1 -> Product/1
  Bus Selector/3 -> Product/2  "<lg_bool>"
  Abs/1 -> CTLST_BETA_ALFA/2

== system kamerol/Aerodynamics/TangentialForceCoefficient/MachRegion2/eoeff ==
  CTDEYODE_M : Lookup_n-D  NumberOfTableDimensions=1  BreakpointsForDimension1=admireDB.aerodata_sym.CTDEYODE.breakpoints.M  BreakpointsForDimension3=[5, 7]  Table=admireDB.aerodata_sym.CTDEYODE.newTable  ExtrapMethod=Clip  InternalRulePriority=Speed  RndMeth=Simplest  InputSameDT=on
  CTDEYODE_M1 : Lookup_n-D  NumberOfTableDimensions=1  BreakpointsForDimension1=admireDB.aerodata_sym.CTDEYODE.breakpoints.M  BreakpointsForDimension3=[5, 7]  Table=admireDB.aerodata_sym.CTDEYODE.newTable  ExtrapMethod=Clip  InternalRulePriority=Speed  RndMeth=Simplest  InputSameDT=on
  Constant : Constant
  Constant1 : Constant  Value=0.4
  Constant2 : Constant  Value=0.5
  Constant3 : Constant
  Sum : Sum  Inputs=-+|
  Sum1 : Sum  Inputs=-+|
  eoefflow : Outport
  eiefflow : Outport  Port=2
  eoeffhigh : Outport  Port=3
  eieffhigh : Outport  Port=4
  wires:
  Sum1/1 -> eieffhigh/1  "eieffhigh"
  CTDEYODE_M1/1 -> eoeffhigh/1, Sum1/1  "eoeffhigh"
  Constant3/1 -> Sum1/2
  Constant2/1 -> CTDEYODE_M1/1
  Constant1/1 -> CTDEYODE_M/1
  Constant/1 -> Sum/2
  CTDEYODE_M/1 -> Sum/1, eoefflow/1  "eoefflow"
  Sum/1 -> eiefflow/1  "eiefflow"

== system kamerol/Aerodynamics/TangentialForceCoefficient/MachRegion3/Ctalfa ==
  in_bus : Inport
  Bus Selector : BusSelector  OutputSignals=AeroIn_Bus.angleOfAttack_deg,AeroIn_Bus.mach_nd
  CTMA_M_ALFA : Lookup_n-D  BreakpointsForDimension1=admireDB.aerodata_sym.CTMA.breakpoints.ALFA  BreakpointsForDimension2=admireDB.aerodata_sym.CTMA.breakpoints.M  BreakpointsForDimension3=[5, 7]  Table=admireDB.aerodata_sym.CTMA.newTable  ExtrapMethod=Clip  InternalRulePriority=Speed  RndMeth=Simplest  InputSameDT=on
      settings: InputPortMap=u0,u1
  Ctalfa : Outport
  wires:
  CTMA_M_ALFA/1 -> Ctalfa/1
  Bus Selector/2 -> CTMA_M_ALFA/2  "<mach_nd>"
  Bus Selector/1 -> CTMA_M_ALFA/1  "<angleOfAttack_deg>"
  in_bus/1 -> Bus Selector/1

== system kamerol/Aerodynamics/TangentialForceCoefficient/MachRegion3/Ctbasic ==
  in_bus : Inport
  Bus Selector : BusSelector  OutputSignals=AeroIn_Bus.mach_nd,AeroIn_Bus.altitude_m
  CTH_H_M : Lookup_n-D  BreakpointsForDimension1=admireDB.aerodata_sym.CTH.breakpoints.M  BreakpointsForDimension2=admireDB.aerodata_sym.CTH.breakpoints.H  BreakpointsForDimension3=[5, 7]  Table=admireDB.aerodata_sym.CTH.newTable  ExtrapMethod=Clip  InternalRulePriority=Speed  RndMeth=Simplest  InputSameDT=on
      settings: InputPortMap=u0,u1
  CTZERO_M : Lookup_n-D  NumberOfTableDimensions=1  BreakpointsForDimension1=admireDB.aerodata_sym.CTZERO.breakpoints.M  BreakpointsForDimension3=[5, 7]  Table=admireDB.aerodata_sym.CTZERO.newTable  ExtrapMethod=Clip  InternalRulePriority=Speed  RndMeth=Simplest  InputSameDT=on
  Constant : Constant  Value=1/1000
  Product : Product
  Sum1 : Sum  Inputs=|++
  Ctbasic : Outport
  wires:
  Sum1/1 -> Ctbasic/1
  in_bus/1 -> Bus Selector/1  "in_bus"
  Bus Selector/1 -> CTZERO_M/1, CTH_H_M/1  "<mach_nd>"
  CTZERO_M/1 -> Sum1/1
  Product/1 -> CTH_H_M/2
  Bus Selector/2 -> Product/1  "<altitude_m>"
  Constant/1 -> Product/2
  CTH_H_M/1 -> Sum1/2

== system kamerol/Aerodynamics/TangentialForceCoefficient/MachRegion3/Ctbeta ==
  Constant : Constant  Value=0
  Ctbeta : Outport
  wires:
  Constant/1 -> Ctbeta/1

== system kamerol/Aerodynamics/TangentialForceCoefficient/MachRegion3/Ctda ==
  in_bus : Inport
  Abs : Abs
  Abs1 : Abs
  Bus Selector : BusSelector  OutputSignals=AeroIn_Bus.mach_nd,AeroIn_Bus.dAI,eieff,AeroIn_Bus.dAY,eoeff
  CTDAM_DA_M : Lookup_n-D  BreakpointsForDimension1=admireDB.aerodata_sym.CTDAM.breakpoints.M  BreakpointsForDimension2=admireDB.aerodata_sym.CTDAM.breakpoints.DA  BreakpointsForDimension3=[5, 7]  Table=admireDB.aerodata_sym.CTDAM.newTable  ExtrapMethod=Clip  InternalRulePriority=Speed  RndMeth=Simplest  InputSameDT=on
      settings: InputPortMap=u0,u1
  CTDAM_DA_M1 : Lookup_n-D  BreakpointsForDimension1=admireDB.aerodata_sym.CTDAM.breakpoints.M  BreakpointsForDimension2=admireDB.aerodata_sym.CTDAM.breakpoints.DA  BreakpointsForDimension3=[5, 7]  Table=admireDB.aerodata_sym.CTDAM.newTable  ExtrapMethod=Clip  InternalRulePriority=Speed  RndMeth=Simplest  InputSameDT=on
      settings: InputPortMap=u0,u1
  Product : Product
  Product1 : Product
  Sum : Sum  Inputs=|++
  Ctda : Outport
  wires:
  Sum/1 -> Ctda/1
  Product1/1 -> Sum/2
  Product/1 -> Sum/1
  Bus Selector/5 -> Product1/2  "<eoeff>"
  CTDAM_DA_M1/1 -> Product1/1
  Abs1/1 -> CTDAM_DA_M1/2
  Bus Selector/4 -> Abs1/1  "<dAY>"
  CTDAM_DA_M/1 -> Product/1
  Bus Selector/3 -> Product/2  "<eieff>"
  Abs/1 -> CTDAM_DA_M/2
  Bus Selector/1 -> CTDAM_DA_M/1, CTDAM_DA_M1/1  "<mach_nd>"
  Bus Selector/2 -> Abs/1  "<dAI>"
  in_bus/1 -> Bus Selector/1

== system kamerol/Aerodynamics/TangentialForceCoefficient/MachRegion3/Ctdedn ==
  Constant : Constant  Value=0
  Ctdedn : Outport
  wires:
  Constant/1 -> Ctdedn/1

== system kamerol/Aerodynamics/TangentialForceCoefficient/MachRegion3/Ctdei ==
  in_bus : Inport
  Bus Selector : BusSelector  OutputSignals=AeroIn_Bus.angleOfAttack_deg,AeroIn_Bus.dEI,AeroIn_Bus.mach_nd,eieff
  CTMDEA_ALFA_DE_M : Lookup_n-D  NumberOfTableDimensions=3  BreakpointsForDimension1=admireDB.aerodata_sym.CTMDEA.breakpoints.ALFA  BreakpointsForDimension2=admireDB.aerodata_sym.CTMDEA.breakpoints.DE  BreakpointsForDimension3=admireDB.aerodata_sym.CTMDEA.breakpoints.M  Table=admireDB.aerodata_sym.CTMDEA.newTable  ExtrapMethod=Clip  InternalRulePriority=Speed  RndMeth=Simplest  InputSameDT=on
      settings: InputPortMap=u0,u1,u2
  Product1 : Product
  Ctdei : Outport
  wires:
  Product1/1 -> Ctdei/1
  Bus Selector/4 -> Product1/2  "<eieff>"
  Bus Selector/3 -> CTMDEA_ALFA_DE_M/3  "<mach_nd>"
  Bus Selector/2 -> CTMDEA_ALFA_DE_M/2  "<dEI>"
  Bus Selector/1 -> CTMDEA_ALFA_DE_M/1  "<angleOfAttack_deg>"
  in_bus/1 -> Bus Selector/1
  CTMDEA_ALFA_DE_M/1 -> Product1/1

== system kamerol/Aerodynamics/TangentialForceCoefficient/MachRegion3/Ctdey ==
  in_bus : Inport
  Bus Selector : BusSelector  OutputSignals=AeroIn_Bus.angleOfAttack_deg,AeroIn_Bus.dEY,AeroIn_Bus.mach_nd,eoeff
  CTMDEA_ALFA_DE_M : Lookup_n-D  NumberOfTableDimensions=3  BreakpointsForDimension1=admireDB.aerodata_sym.CTMDEA.breakpoints.ALFA  BreakpointsForDimension2=admireDB.aerodata_sym.CTMDEA.breakpoints.DE  BreakpointsForDimension3=admireDB.aerodata_sym.CTMDEA.breakpoints.M  Table=admireDB.aerodata_sym.CTMDEA.newTable  ExtrapMethod=Clip  InternalRulePriority=Speed  RndMeth=Simplest  InputSameDT=on
      settings: InputPortMap=u0,u1,u2
  Product1 : Product
  Ctdey : Outport
  wires:
  Product1/1 -> Ctdey/1
  Bus Selector/4 -> Product1/2  "<eoeff>"
  Bus Selector/3 -> CTMDEA_ALFA_DE_M/3  "<mach_nd>"
  Bus Selector/2 -> CTMDEA_ALFA_DE_M/2  "<dEY>"
  Bus Selector/1 -> CTMDEA_ALFA_DE_M/1  "<angleOfAttack_deg>"
  in_bus/1 -> Bus Selector/1
  CTMDEA_ALFA_DE_M/1 -> Product1/1

== system kamerol/Aerodynamics/TangentialForceCoefficient/MachRegion3/Ctdle ==
  in_bus : Inport
  Bus Selector : BusSelector  OutputSignals=AeroIn_Bus.angleOfAttack_deg,AeroIn_Bus.lef_deg,AeroIn_Bus.mach_nd
  CTMDLEA_ALFA_DLE_M : Lookup_n-D  NumberOfTableDimensions=3  BreakpointsForDimension1=admireDB.aerodata_sym.CTMDLEA.breakpoints.ALFA  BreakpointsForDimension2=admireDB.aerodata_sym.CTMDLEA.breakpoints.DLE  BreakpointsForDimension3=admireDB.aerodata_sym.CTMDLEA.breakpoints.M  Table=admireDB.aerodata_sym.CTMDLEA.newTable  ExtrapMethod=Clip  InternalRulePriority=Speed  RndMeth=Simplest  InputSameDT=on
      settings: InputPortMap=u0,u1,u2
  Ctdle : Outport
  wires:
  Bus Selector/1 -> CTMDLEA_ALFA_DLE_M/1  "<angleOfAttack_deg>"
  Bus Selector/3 -> CTMDLEA_ALFA_DLE_M/3  "<mach_nd>"
  Bus Selector/2 -> CTMDLEA_ALFA_DLE_M/2  "<lef_deg>"
  CTMDLEA_ALFA_DLE_M/1 -> Ctdle/1
  in_bus/1 -> Bus Selector/1

== system kamerol/Aerodynamics/TangentialForceCoefficient/MachRegion3/Ctdn ==
  in_bus : Inport
  Bus Selector : BusSelector  OutputSignals=AeroIn_Bus.angleOfAttack_deg,AeroIn_Bus.dN,AeroIn_Bus.mach_nd
  CTMDNA_ALFA_DN_M : Lookup_n-D  NumberOfTableDimensions=3  BreakpointsForDimension1=admireDB.aerodata_sym.CTMDNA.breakpoints.ALFA  BreakpointsForDimension2=admireDB.aerodata_sym.CTMDNA.breakpoints.DN  BreakpointsForDimension3=admireDB.aerodata_sym.CTMDNA.breakpoints.M  Table=admireDB.aerodata_sym.CTMDNA.newTable  ExtrapMethod=Clip  InternalRulePriority=Speed  RndMeth=Simplest  InputSameDT=on
      settings: InputPortMap=u0,u1,u2
  Ctdn : Outport
  wires:
  Bus Selector/1 -> CTMDNA_ALFA_DN_M/1  "<angleOfAttack_deg>"
  Bus Selector/2 -> CTMDNA_ALFA_DN_M/2  "<dN>"
  Bus Selector/3 -> CTMDNA_ALFA_DN_M/3  "<mach_nd>"
  in_bus/1 -> Bus Selector/1
  CTMDNA_ALFA_DN_M/1 -> Ctdn/1

== system kamerol/Aerodynamics/TangentialForceCoefficient/MachRegion3/Ctdr ==
  in_bus : Inport
  Abs : Abs
  Bus Selector : BusSelector  OutputSignals=AeroIn_Bus.mach_nd,AeroIn_Bus.rud_deg
  CTMDR_DR_M : Lookup_n-D  BreakpointsForDimension1=admireDB.aerodata_sym.CTMDR.breakpoints.M  BreakpointsForDimension2=admireDB.aerodata_sym.CTMDR.breakpoints.DR  BreakpointsForDimension3=[5, 7]  Table=admireDB.aerodata_sym.CTMDR.newTable  ExtrapMethod=Clip  InternalRulePriority=Speed  RndMeth=Simplest  InputSameDT=on
      settings: InputPortMap=u0,u1
  Ctdr : Outport
  wires:
  Abs/1 -> CTMDR_DR_M/2
  Bus Selector/1 -> CTMDR_DR_M/1  "<mach_nd>"
  Bus Selector/2 -> Abs/1  "<rud_deg>"
  in_bus/1 -> Bus Selector/1
  CTMDR_DR_M/1 -> Ctdr/1

== system kamerol/Aerodynamics/TangentialForceCoefficient/MachRegion3/Cthigh ==
  Constant : Constant  Value=0
  Cthigh : Outport
  wires:
  Constant/1 -> Cthigh/1

== system kamerol/Aerodynamics/TangentialForceCoefficient/MachRegion3/Ctlg ==
  in_bus : Inport
  Abs : Abs
  Bus Selector : BusSelector  OutputSignals=AeroIn_Bus.angleOfAttack_deg,AeroIn_Bus.angleOfSideslip_deg,AeroIn_Bus.lg_bool
  CTLST_BETA_ALFA : Lookup_n-D  BreakpointsForDimension1=admireDB.aerodata_sym.CTLST.breakpoints.ALFA  BreakpointsForDimension2=admireDB.aerodata_sym.CTLST.breakpoints.BETA  BreakpointsForDimension3=[5, 7]  Table=admireDB.aerodata_sym.CTLST.newTable  ExtrapMethod=Clip  InternalRulePriority=Speed  RndMeth=Simplest  InputSameDT=on
      settings: InputPortMap=u0,u1
  Product : Product  Inputs=**
  Ctlg : Outport
  wires:
  Abs/1 -> CTLST_BETA_ALFA/2
  Bus Selector/3 -> Product/2  "<lg_bool>"
  CTLST_BETA_ALFA/1 -> Product/1
  in_bus/1 -> Bus Selector/1
  Bus Selector/2 -> Abs/1  "<angleOfSideslip_deg>"
  Bus Selector/1 -> CTLST_BETA_ALFA/1  "<angleOfAttack_deg>"
  Product/1 -> Ctlg/1

== system kamerol/Aerodynamics/TangentialForceCoefficient/MachRegion3/eoeff ==
  AeroIn_Bus : Inport
  Bus Selector : BusSelector  OutputSignals=mach_nd
  CTDEYODE_M : Lookup_n-D  NumberOfTableDimensions=1  BreakpointsForDimension1=admireDB.aerodata_sym.CTDEYODE.breakpoints.M  BreakpointsForDimension3=[5, 7]  Table=admireDB.aerodata_sym.CTDEYODE.newTable  ExtrapMethod=Clip  InternalRulePriority=Speed  RndMeth=Simplest  InputSameDT=on
  Constant : Constant
  Sum : Sum  Inputs=-+|
  eoeff : Outport
  eieff : Outport  Port=2
  wires:
  Sum/1 -> eieff/1
  CTDEYODE_M/1 -> eoeff/1, Sum/1
  Constant/1 -> Sum/2
  Bus Selector/1 -> CTDEYODE_M/1  "<mach_nd>"
  AeroIn_Bus/1 -> Bus Selector/1

== system kamerol/Aerodynamics/YawMomentCoefficient/MachRegion1/Cymbasic ==
  in_bus : Inport
  Bus Selector : BusSelector  OutputSignals=AeroIn_Bus.angleOfAttack_deg
  Cymbasic_ : Subsystem
  Cymbasic : Outport
  wires:
  Cymbasic_/1(Cymbasic) -> Cymbasic/1
  Bus Selector/1 -> Cymbasic_/1(angleOfAttack_deg)  "<angleOfAttack_deg>"
  in_bus/1 -> Bus Selector/1  "in_bus"

== system kamerol/Aerodynamics/YawMomentCoefficient/MachRegion1/Cymbcai ==
  in_bus : Inport
  Bus Selector : BusSelector  OutputSignals=AeroIn_Bus.cai,AeroIn_Bus.angleOfAttack_deg,AeroIn_Bus.angleOfSideslip_deg
  Cymbcai_ : Subsystem
  Cymbcai : Outport
  wires:
  Bus Selector/3 -> Cymbcai_/3(angleOfSideslip_deg)  "<angleOfSideslip_deg>"
  Bus Selector/2 -> Cymbcai_/2(angleOfAttack_deg)  "<angleOfAttack_deg>"
  Bus Selector/1 -> Cymbcai_/1(CAI)  "<cai>"
  in_bus/1 -> Bus Selector/1  "in_bus"
  Cymbcai_/1(Cymbcai) -> Cymbcai/1

== system kamerol/Aerodynamics/YawMomentCoefficient/MachRegion1/Cymbde ==
  in_bus : Inport
  Bus Selector : BusSelector  OutputSignals=AeroIn_Bus.angleOfAttack_deg,AeroIn_Bus.dEI,AeroIn_Bus.angleOfSideslip_deg,AeroIn_Bus.dEY,eieff,eoeff
  Cymbde_ : Subsystem
  Cymbde : Outport
  wires:
  Bus Selector/6 -> Cymbde_/6(eoeff)  "<eoeff>"
  Bus Selector/5 -> Cymbde_/5(eieff)  "<eieff>"
  Bus Selector/4 -> Cymbde_/4(dEY)  "<dEY>"
  Bus Selector/3 -> Cymbde_/3(angleOfSideslip_deg)  "<angleOfSideslip_deg>"
  Bus Selector/2 -> Cymbde_/2(dEI)  "<dEI>"
  Bus Selector/1 -> Cymbde_/1(angleOfAttack_deg)  "<angleOfAttack_deg>"
  Cymbde_/1(Cymbde) -> Cymbde/1
  in_bus/1 -> Bus Selector/1  "in_bus"

== system kamerol/Aerodynamics/YawMomentCoefficient/MachRegion1/Cymbdle ==
  in_bus : Inport
  Bus Selector : BusSelector  OutputSignals=AeroIn_Bus.angleOfAttack_deg,AeroIn_Bus.dEI,AeroIn_Bus.angleOfSideslip_deg,AeroIn_Bus.lef_deg,AeroIn_Bus.dEY,eieff,eoeff
  Cymbdle_ : Subsystem
  Cymbdle : Outport
  wires:
  Bus Selector/2 -> Cymbdle_/2(dEI)  "<dEI>"
  Bus Selector/1 -> Cymbdle_/1(angleOfAttack_deg)  "<angleOfAttack_deg>"
  Bus Selector/3 -> Cymbdle_/3(angleOfSideslip_deg)  "<angleOfSideslip_deg>"
  Bus Selector/4 -> Cymbdle_/4(dLE)  "<lef_deg>"
  Bus Selector/5 -> Cymbdle_/5(dEY)  "<dEY>"
  Bus Selector/6 -> Cymbdle_/6(eieff)  "<eieff>"
  Bus Selector/7 -> Cymbdle_/7(eoeff)  "<eoeff>"
  Cymbdle_/1(Cymbdle) -> Cymbdle/1
  in_bus/1 -> Bus Selector/1  "in_bus"

== system kamerol/Aerodynamics/YawMomentCoefficient/MachRegion1/Cymbdn ==
  in_bus : Inport
  Bus Selector : BusSelector  OutputSignals=AeroIn_Bus.angleOfAttack_deg,AeroIn_Bus.dN,AeroIn_Bus.angleOfSideslip_deg
  Cymbdn_ : Subsystem
  Cymbdn : Outport
  wires:
  Bus Selector/1 -> Cymbdn_/1(angleOfAttack_deg)  "<angleOfAttack_deg>"
  Bus Selector/3 -> Cymbdn_/3(angleOfSideslip_deg)  "<angleOfSideslip_deg>"
  Bus Selector/2 -> Cymbdn_/2(dN)  "<dN>"
  in_bus/1 -> Bus Selector/1  "in_bus"
  Cymbdn_/1(Cymbdn) -> Cymbdn/1

== system kamerol/Aerodynamics/YawMomentCoefficient/MachRegion1/Cymbeta ==
  in_bus : Inport
  Bus Selector : BusSelector  OutputSignals=AeroIn_Bus.angleOfSideslip_deg,AeroIn_Bus.angleOfAttack_deg,AeroIn_Bus.qacorr,AeroIn_Bus.mach_nd
  Cymbeta_ : Subsystem
  Cymbeta : Outport
  wires:
  Bus Selector/4 -> Cymbeta_/4(mach_nd)  "<mach_nd>"
  Bus Selector/3 -> Cymbeta_/3(qacorr)  "<qacorr>"
  Bus Selector/2 -> Cymbeta_/2(angleOfAttack_deg)  "<angleOfAttack_deg>"
  Bus Selector/1 -> Cymbeta_/1(angleOfSideslip_deg)  "<angleOfSideslip_deg>"
  in_bus/1 -> Bus Selector/1  "in_bus"
  Cymbeta_/1(Cymbeta) -> Cymbeta/1

== system kamerol/Aerodynamics/YawMomentCoefficient/MachRegion1/Cymbetad ==
  in_bus : Inport
  Bus Selector : BusSelector  OutputSignals=AeroIn_Bus.angleOfAttack_deg,AeroIn_Bus.betad
  Cymbetad_ : Subsystem
  Cymbetad : Outport
  wires:
  Bus Selector/1 -> Cymbetad_/1(angleOfAttack_deg)  "<angleOfAttack_deg>"
  Bus Selector/2 -> Cymbetad_/2(betad)  "<betad>"
  Cymbetad_/1(Cymbetad) -> Cymbetad/1
  in_bus/1 -> Bus Selector/1  "in_bus"

== system kamerol/Aerodynamics/YawMomentCoefficient/MachRegion1/Cymblg ==
  in_bus : Inport
  Bus Selector : BusSelector  OutputSignals=AeroIn_Bus.angleOfSideslip_deg,AeroIn_Bus.lg_bool,AeroIn_Bus.angleOfAttack_deg
  Cymblg_ : Subsystem
  Cymblg : Outport
  wires:
  Bus Selector/3 -> Cymblg_/3(angleOfAttack_deg)  "<angleOfAttack_deg>"
  Bus Selector/1 -> Cymblg_/1(angleOfSideslip_deg)  "<angleOfSideslip_deg>"
  Bus Selector/2 -> Cymblg_/2(dLG)  "<lg_bool>"
  Cymblg_/1(Cymblg) -> Cymblg/1
  in_bus/1 -> Bus Selector/1  "in_bus"

== system kamerol/Aerodynamics/YawMomentCoefficient/MachRegion1/Cymdai ==
  in_bus : Inport
  Bus Selector : BusSelector  OutputSignals=AeroIn_Bus.dAI,AeroIn_Bus.angleOfAttack_deg,AeroIn_Bus.dEI,eieff,AeroIn_Bus.qacorr,AeroIn_Bus.mach_nd
  Cymdai_ : Subsystem
  Cymdai : Outport
  wires:
  Bus Selector/1 -> Cymdai_/1(dAI)  "<dAI>"
  Bus Selector/2 -> Cymdai_/2(angleOfAttack_deg)  "<angleOfAttack_deg>"
  Bus Selector/3 -> Cymdai_/3(dEI)  "<dEI>"
  Bus Selector/4 -> Cymdai_/4(eieff)  "<eieff>"
  Bus Selector/5 -> Cymdai_/5(qacorr)  "<qacorr>"
  Bus Selector/6 -> Cymdai_/6(mach_nd)  "<mach_nd>"
  Cymdai_/1(Cymdai) -> Cymdai/1
  in_bus/1 -> Bus Selector/1  "in_bus"

== system kamerol/Aerodynamics/YawMomentCoefficient/MachRegion1/Cymdaib ==
  in_bus : Inport
  Bus Selector : BusSelector  OutputSignals=AeroIn_Bus.angleOfAttack_deg,AeroIn_Bus.dAI,AeroIn_Bus.angleOfSideslip_deg,eieff
  Cymdaib_ : Subsystem
  Cymdaib : Outport
  wires:
  Bus Selector/4 -> Cymdaib_/4(eieff)  "<eieff>"
  Bus Selector/3 -> Cymdaib_/3(angleOfSideslip_deg)  "<angleOfSideslip_deg>"
  Bus Selector/2 -> Cymdaib_/2(dAI)  "<dAI>"
  Bus Selector/1 -> Cymdaib_/1(angleOfAttack_deg)  "<angleOfAttack_deg>"
  Cymdaib_/1(Cymdaib) -> Cymdaib/1
  in_bus/1 -> Bus Selector/1  "in_bus"
